simulink model "triggersubsystem"  (R2018a)
settings: Solver=FixedStepDiscrete  StartTime=0.0  StopTime=10.0  RelTol=1e-3
libraries: simulink x1
settings Model: Creator=SONY  LastModifiedBy=SONY

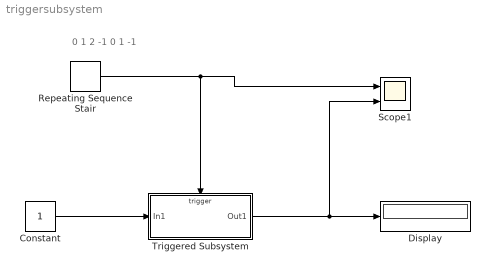
== system triggersubsystem ==
  note: 0 1 2 -1 0 1 -1
  Constant : Constant
  Display : Display
  Repeating Sequence Stair : simulink/Sources/Repeating Sequence Stair  OutValues=[0 1 2 -1 0 1 -1].'  tsamp=-1  OutMin=[]  OutMax=[]  OutDataTypeStr=double  OutputDataTypeScalingMode=double  OutDataType=fixdt(0,8)  ConRadixGroup=Best Precision: Vector-wise  OutScaling=2^-12
  Scope1 : Scope  NumInputPorts=2
  Triggered Subsystem : Subsystem  TreatAsAtomicUnit=on
  wires:
  Triggered Subsystem/1(Out1) -> Scope1/2, Display/1
  Constant/1 -> Triggered Subsystem/1(In1)
  Repeating Sequence Stair/1 -> Scope1/1, Triggered Subsystem/Trigger

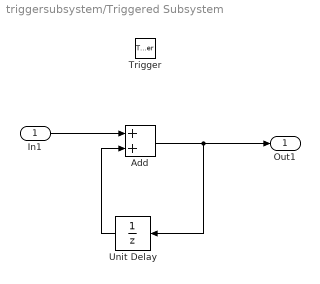
== system triggersubsystem/Triggered Subsystem ==
  In1 : Inport
  Trigger : TriggerPort  TriggerType=either  VariantControl=Variant
  Add : Sum
  Unit Delay : UnitDelay  SampleTime=-1
  Out1 : Outport
  wires:
  In1/1 -> Add/1
  Add/1 -> Unit Delay/1, Out1/1
  Unit Delay/1 -> Add/2
